simulink model "torque_pi_controller_incremental_algorithm"  (R2023b)
settings: Solver=VariableStepAuto  StartTime=0.0  StopTime=10.0  RelTol=1e-5
values from neighbouring files (symbols this model uses):
  K = 1.32    [torque_PI_integral_algorithm.m]    (also in torque_PI_tuning.m; torque_model.m)
  Kp = 0.45966    [torque_PI_integral_algorithm.m]
  Ti = 1/(Ki/Kp)    (= 0.000676567559611)    [torque_PI_integral_algorithm.m]
  Ts = 0.005    [torque_PI_integral_algorithm.m]    (also in torque_PI_tuning.m)
undefined symbols (not defined in the file or in its folder): DiscIntNeverNeededParam
settings Model: Creator=paoli  LastModifiedBy=paoli

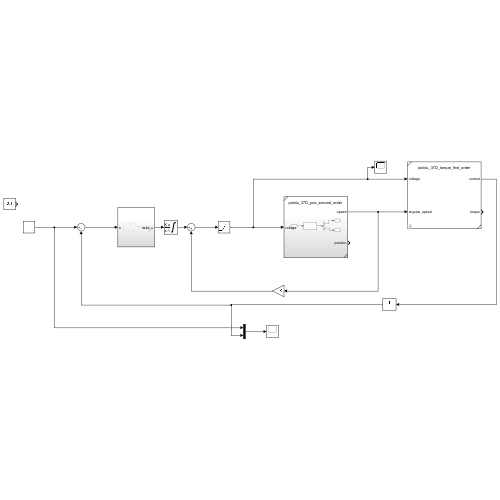
[thumbnail: Simulink's stored preview of the top-level diagram]
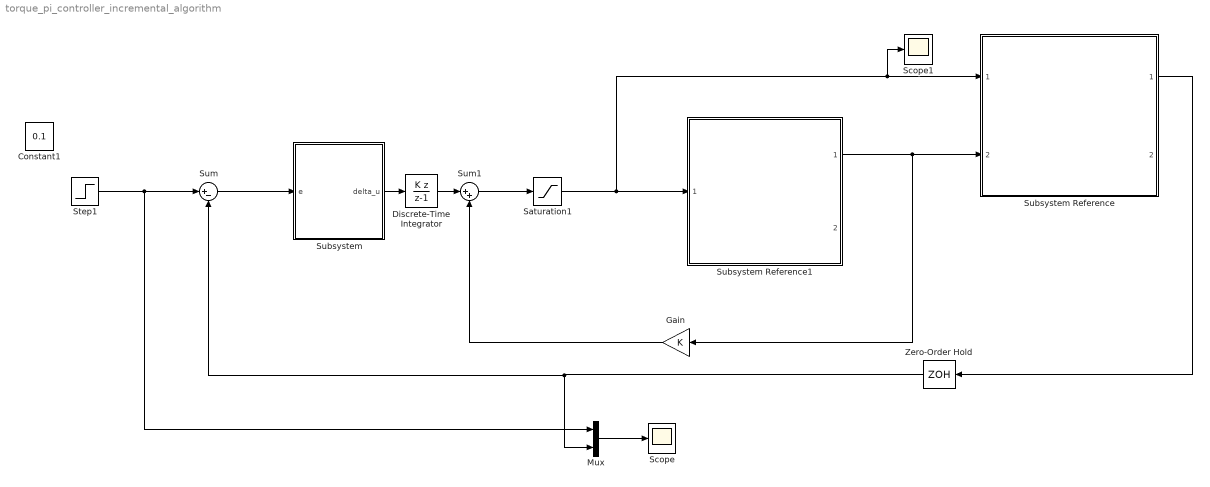
== system torque_pi_controller_incremental_algorithm ==
  Constant1 : Constant  Value=0.1
  Discrete-Time Integrator : DiscreteIntegrator  IntegratorMethod=Accumulation: Backward Euler  SampleTime=-1  LimitOutput=on  UpperSaturationLimit=12  LowerSaturationLimit=-12  ICPrevOutput=DiscIntNeverNeededParam  ICPrevScaledInput=DiscIntNeverNeededParam
  Gain : Gain  Gain=K
  Mux : Mux  Inputs=2
  Saturation1 : Saturate  UpperLimit=12  LowerLimit=-12
  Scope : Scope
  Scope1 : Scope
  Step1 : Step  Time=3  Before=1  After=0  SampleTime=0
  Subsystem : Subsystem
  Subsystem Reference : Subsystem  ReferencedSubsystem=pololu_37D_torque_first_order  L=2.3e-3  R=2.1  K=1.32
  Subsystem Reference1 : Subsystem  ReferencedSubsystem=pololu_37D_pos_second_order
  Sum : Sum  Inputs=|+-
  Sum1 : Sum  Inputs=|++
  Zero-Order Hold : ZeroOrderHold  SampleTime=Ts
  wires:
  Subsystem Reference/1 -> Zero-Order Hold/1
  Step1/1 -> Mux/1, Sum/1
  Mux/1 -> Scope/1
  Subsystem Reference1/1 -> Gain/1, Subsystem Reference/2
  Sum1/1 -> Saturation1/1
  Saturation1/1 -> Scope1/1, Subsystem Reference/1, Subsystem Reference1/1
  Sum/1 -> Subsystem/1(e)
  Subsystem/1(delta_u) -> Discrete-Time Integrator/1
  Discrete-Time Integrator/1 -> Sum1/1
  Gain/1 -> Sum1/2
  Zero-Order Hold/1 -> Mux/2, Sum/2

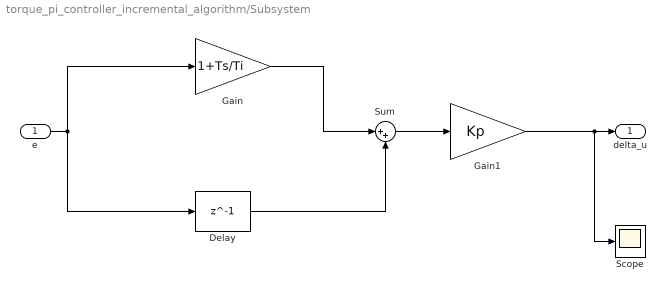
== system torque_pi_controller_incremental_algorithm/Subsystem ==
  e : Inport  SampleTime=Ts
  Delay : Delay  DelayLength=1  InitialCondition=0  UseCircularBuffer=on
  Gain : Gain  Gain=1+Ts/Ti
  Gain1 : Gain  Gain=Kp
  Scope : Scope
  Sum : Sum  Inputs=|++
  delta_u : Outport  SampleTime=Ts
  wires:
  e/1 -> Delay/1, Gain/1
  Delay/1 -> Sum/2
  Gain/1 -> Sum/1
  Sum/1 -> Gain1/1
  Gain1/1 -> Scope/1, delta_u/1
